simulink model "exsim2model"  (Simulink 7.2)
settings: Solver=ode45  StartTime=0.0  StopTime=tf  FixedStep=T  RelTol=1e-3
values from neighbouring files (symbols this model uses):
  a = 2*w0    (= 2)    [exsim2script.m]
  b = w0/2    (= 0.5)    [exsim2script.m]
  J = 1    [exsim2script.m]
  kc = 2*J*w0^2/kp    (= 2)    [exsim2script.m]
  kp = 1    [exsim2script.m]
  T = 0:SAMPLES-1    [discrete.m]    (also in exsim2script.m = 1.08)
settings Model: Creator=hcf2k  LastModifiedBy=hcf2k  CovModelRefEnable=off
settings DataIOCC: SaveFormat=StructureWithTime
settings OptimizationCC: ExpressionDepthLimit=128
settings DebuggingCC: UnderspecifiedInitializationDetection=Simplified  MergeDetectMultiDrivingBlocksExec=error  SolverPrmCheckMsg=none  FcnCallInpInsideContextMsg=Enable All  StateNameClashWarn=none  StrictBusMsg=ErrorLevel1
settings HardwareCC: ProdIntDivRoundTo=Zero  ProdEndianess=LittleEndian  ProdHWDeviceType=Specified
settings CodeAppCC: CustomSymbolStrType=$N$R$M_T
settings GRTTargetCC: TargetFunctionLibrary=C89/C90 (ANSI)

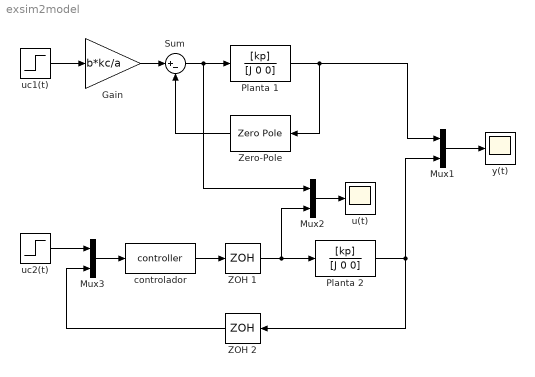
== system exsim2model ==
  Gain : Gain  Gain=b*kc/a
  Mux1 : Mux  Inputs=2
  Mux2 : Mux  Inputs=2
  Mux3 : Mux  Inputs=2
  Planta 1 : TransferFcn  Numerator=[kp]  Denominator=[J 0 0]
  Planta 2 : TransferFcn  Numerator=[kp]  Denominator=[J 0 0]
  Sum : Sum  Inputs=|+-
  ZOH 1 : ZeroOrderHold  SampleTime=T
  ZOH 2 : ZeroOrderHold  Orientation=left  SampleTime=T
  Zero-Pole : ZeroPole  Orientation=left  Zeros=[-b]  Poles=[-a]  Gain=[kc]
  controlador : MATLABFcn  MATLABFcn=controller  OutputDimensions=1
  u(t) : Scope
      settings: TimeRange=auto  MaxDataPoints=5000  SaveName=u  YMin=-0.40773  YMax=0.60086  SampleTime=-1  DataFormat=Array
  uc1(t) : Step  Time=0  SampleTime=0
  uc2(t) : Step  Time=0  SampleTime=T
  y(t) : Scope
      settings: TimeRange=auto  MaxDataPoints=5000  SaveName=y  YMin=-0.15943  YMax=1.43486  SampleTime=-1  DataFormat=Array
  wires:
  Planta 1/1 -> Mux1/1, Zero-Pole/1
  Mux1/1 -> y(t)/1
  Mux2/1 -> u(t)/1
  Planta 2/1 -> ZOH 2/1, Mux1/2
  controlador/1 -> ZOH 1/1
  ZOH 1/1 -> Planta 2/1, Mux2/2
  Sum/1 -> Planta 1/1, Mux2/1
  Mux3/1 -> controlador/1
  Gain/1 -> Sum/1
  Zero-Pole/1 -> Sum/2
  ZOH 2/1 -> Mux3/2
  uc2(t)/1 -> Mux3/1
  uc1(t)/1 -> Gain/1
